simulink model "Downstream"  (R2023b)
settings: Solver=FixedStepDiscrete  StartTime=0.0  StopTime=inf  FixedStep=.05  RelTol=1e-3
model workspace (MAT data in the model file):
  SL_ROS_VariableLengthArrays_MaxSizes.CommonInfo.ArrayTruncateAction = 'EmitWarning'
  SL_ROS_VariableLengthArrays_MaxSizes.MsgTypeMap = containers.Map
  SL_ROS_VariableLengthArrays_MaxSizes.MsgTypeMap.serialization.keys = {'sensor_msgs/Image', 'sensor_msgs/PointCloud2'}
  SL_ROS_VariableLengthArrays_MaxSizes.MsgTypeMap.serialization.values{1}(1).PropertyName = 'Data'
  SL_ROS_VariableLengthArrays_MaxSizes.MsgTypeMap.serialization.values{1}(1).DataType = 'uint8'
  SL_ROS_VariableLengthArrays_MaxSizes.MsgTypeMap.serialization.values{1}(1).MaxLength = 1920000
  SL_ROS_VariableLengthArrays_MaxSizes.MsgTypeMap.serialization.values{1}(2).PropertyName = 'Encoding'
  SL_ROS_VariableLengthArrays_MaxSizes.MsgTypeMap.serialization.values{1}(2).DataType = 'uint8'
  SL_ROS_VariableLengthArrays_MaxSizes.MsgTypeMap.serialization.values{1}(2).MaxLength = 128
  SL_ROS_VariableLengthArrays_MaxSizes.MsgTypeMap.serialization.values{2}(1).PropertyName = 'Data'
  SL_ROS_VariableLengthArrays_MaxSizes.MsgTypeMap.serialization.values{2}(1).DataType = 'uint8'
  SL_ROS_VariableLengthArrays_MaxSizes.MsgTypeMap.serialization.values{2}(1).MaxLength = 1920000
  SL_ROS_VariableLengthArrays_MaxSizes.MsgTypeMap.serialization.values{2}(2).PropertyName = 'Fields'
  SL_ROS_VariableLengthArrays_MaxSizes.MsgTypeMap.serialization.values{2}(2).DataType = 'sensor_msgs/PointField'
  SL_ROS_VariableLengthArrays_MaxSizes.MsgTypeMap.serialization.values{2}(2).MaxLength = 16
  SL_ROS_VariableLengthArrays_MaxSizes.MsgTypeMap.serialization.uniformity = 0
  SL_ROS_VariableLengthArrays_MaxSizes.MsgTypeMap.serialization.keyType = 'char'
  SL_ROS_VariableLengthArrays_MaxSizes.MsgTypeMap.serialization.valueType = 'any'
undefined symbols (not defined in the file): brake, gear, hand_brake, manual_gear_shift, reverse, steer, throttle
libraries: ros2lib x3
settings Model: Creator=The MathWorks, Inc.  LastModifiedBy=nikos
settings SolverCC: AlgebraicLoopSolver=TrustRegion
settings DataIOCC: ReturnWorkspaceOutputs=off
settings OptimizationCC: EnhancedBackFolding=on  PassReuseOutputArgsAs=Individual arguments  ZeroExternalMemoryAtStartup=off  ZeroInternalMemoryAtStartup=off  MaxStackSize=64  OptimizeBlockOrder=speed  DifferentSizesBufferReuse=on  OptimizationCustomize=off  EfficientTunableParamExpr=on
settings DebuggingCC: ParameterTunabilityLossMsg=error  UnconnectedInputMsg=warning  UnconnectedOutputMsg=warning  UnconnectedLineMsg=warning  ArithmeticOperatorsInVariantConditions=warning
settings HardwareCC: ProdBitPerLong=64  ProdHWDeviceType=Intel->x86-64 (Linux 64)  UseEmbeddedCoderFeatures=off
settings ModelReferenceCC: EnableRefExpFcnMdlSchedulingChecks=on
settings SFSimCC: SimUseLocalCustomCode=off  MATLABDynamicMemAlloc=off
settings RTWCC: Description=Embedded Coder  SystemTargetFile=ert.tlc  HardwareBoard=Robot Operating System 2 (ROS 2)  TLCOptions="-aInlineSetEventsForThisBaseRateFcn=TLC_FALSE -aSuppressMultiTaskScheduler=TLC_FALSE  -aRateBasedStepFcn=0"  TemplateMakefile=ert_default_tmf  RTWUseLocalCustomCode=off  Toolchain=Colcon Tools  TargetLang=C++
settings CodeAppCC: ForceParamTrailComments=on  IgnoreCustomStorageClasses=off  OperatorAnnotations=on  SimulinkDataObjDesc=on  SFDataObjDesc=on  InsertBlockDesc=on
settings ERTTargetCC: CodeInterfacePackaging=C++ class  SupportNonInlinedSFcns=on

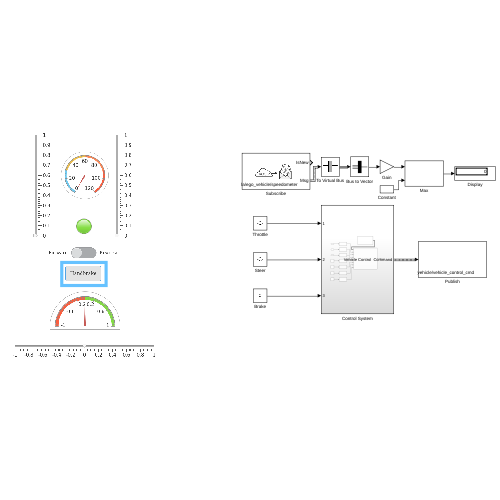
[thumbnail: Simulink's stored preview of the top-level diagram]
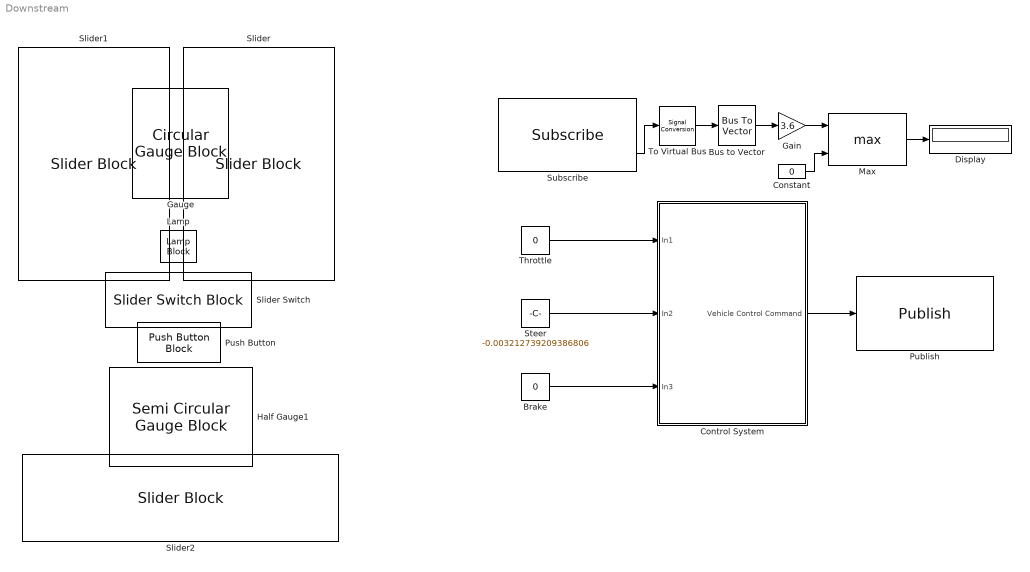
== system Downstream ==
  Brake : Constant  Value=0
  Bus to Vector : BusToVector
  Constant : Constant  Value=0
  Control System : Subsystem
  Display : Display
  Gain : Gain  Gain=3.6
  Gauge : CircularGaugeBlock  LabelPosition=Hide  ScaleMax=120
  Half Gauge1 : SemiCircularGaugeBlock  LabelPosition=Hide  ScaleMin=-1  ScaleMax=1
  Lamp : LampBlock  LabelPosition=Hide
  Max : MinMax  Function=max  Inputs=2
  Publish : ros2lib/Publish  topicSource=Select from ROS network  topic=/carla/ego_vehicle/vehicle_control_cmd  messageType=carla_msgs/CarlaEgoVehicleControl  QOSHistory=Keep last  QOSDepth=1  QOSReliability=Reliable  QOSDurability=Volatile
  Push Button : PushButtonBlock  ButtonText=Handbrake  ButtonType=Latch  IconColor=On  OffValue=0.000000
  Slider : SliderBlock  LabelPosition=Hide  ScaleMax=1
  Slider Switch : SliderSwitchBlock  LabelPosition=Hide
      settings: Values={{'Forward', 'Reverse'}, [0 1]}
  Slider1 : SliderBlock  LabelPosition=Hide  ScaleMax=1
  Slider2 : SliderBlock  LabelPosition=Hide  ScaleMin=-1  ScaleMax=1
  Steer : Constant  Value=-0.003212739209386806
  Subscribe : ros2lib/Subscribe  topicSource=Select from ROS network  topic=/carla/ego_vehicle/speedometer  messageType=std_msgs/Float32  sampleTime=-1  QOSHistory=Keep last  QOSDepth=1  QOSReliability=Reliable  QOSDurability=Volatile
  Throttle : Constant  Value=0
  To Virtual Bus : SignalConversion  ConversionOutput=Virtual bus  OverrideOpt=off
  wires:
  Throttle/1 -> Control System/1(In1)
  Steer/1 -> Control System/2(In2)
  Brake/1 -> Control System/3(In3)
  Control System/1(Vehicle Control Command) -> Publish/1
  Subscribe/2 -> To Virtual Bus/1
  To Virtual Bus/1 -> Bus to Vector/1
  Bus to Vector/1 -> Gain/1
  Gain/1 -> Max/1
  Max/1 -> Display/1
  Constant/1 -> Max/2

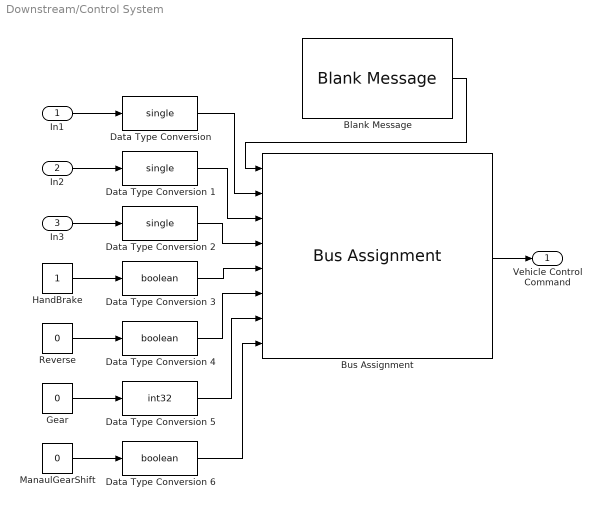
== system Downstream/Control System ==
  In1 : Inport
  In2 : Inport  Port=2
  In3 : Inport  Port=3
  Blank Message : ros2lib/Blank Message  messageClass=Message  entityType=carla_msgs/CarlaEgoVehicleControl  messageType=carla_msgs/CarlaEgoVehicleControl  SampleTime=inf
  Bus Assignment : BusAssignment  AssignedSignals=throttle,steer,brake,hand_brake,reverse,gear,manual_gear_shift
  Data Type Conversion : DataTypeConversion  OutDataTypeStr=single  SaturateOnIntegerOverflow=off  RndMeth=Floor
  Data Type Conversion 1 : DataTypeConversion  OutDataTypeStr=single  SaturateOnIntegerOverflow=off  RndMeth=Floor
  Data Type Conversion 2 : DataTypeConversion  OutDataTypeStr=single  SaturateOnIntegerOverflow=off  RndMeth=Floor
  Data Type Conversion 3 : DataTypeConversion  OutDataTypeStr=boolean  SaturateOnIntegerOverflow=off  RndMeth=Floor
  Data Type Conversion 4 : DataTypeConversion  OutDataTypeStr=boolean  SaturateOnIntegerOverflow=off  RndMeth=Floor
  Data Type Conversion 5 : DataTypeConversion  OutDataTypeStr=int32  SaturateOnIntegerOverflow=off  RndMeth=Floor
  Data Type Conversion 6 : DataTypeConversion  OutDataTypeStr=boolean  SaturateOnIntegerOverflow=off  RndMeth=Floor
  Gear : Constant  Value=0
  HandBrake : Constant
  ManaulGearShift : Constant  Value=0
  Reverse : Constant  Value=0
  Vehicle Control Command : Outport
  wires:
  ManaulGearShift/1 -> Data Type Conversion 6/1
  Data Type Conversion 2/1 -> Bus Assignment/4
  Data Type Conversion 5/1 -> Bus Assignment/7
  Data Type Conversion/1 -> Bus Assignment/2
  Reverse/1 -> Data Type Conversion 4/1
  Data Type Conversion 4/1 -> Bus Assignment/6
  In3/1 -> Data Type Conversion 2/1
  Data Type Conversion 1/1 -> Bus Assignment/3
  In2/1 -> Data Type Conversion 1/1
  In1/1 -> Data Type Conversion/1
  Data Type Conversion 3/1 -> Bus Assignment/5
  Data Type Conversion 6/1 -> Bus Assignment/8
  HandBrake/1 -> Data Type Conversion 3/1
  Blank Message/1 -> Bus Assignment/1
  Bus Assignment/1 -> Vehicle Control Command/1
  Gear/1 -> Data Type Conversion 5/1
